simulink model "untitled"  (R2015a)
settings: Solver=ode45  StartTime=0.0  StopTime=10.0  RelTol=1e-3
settings Model: Creator=TaD  LastModifiedBy=TaD

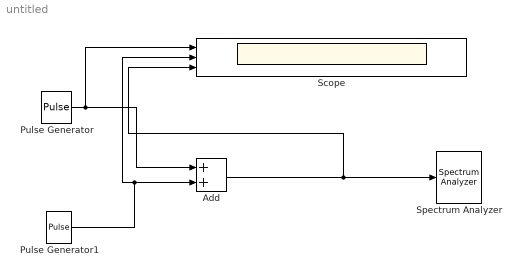
== system untitled ==
  Add : Sum
  Pulse Generator : DiscretePulseGenerator  Amplitude=3  Period=10  PulseWidth=2  VectorParams1D=off
  Pulse Generator1 : DiscretePulseGenerator  PulseType=Time based  Period=10  PulseWidth=5
  Scope : Scope  NumInputPorts=3
      settings: YMin=-5~-5~-5  YMax=5~5~5
  Spectrum Analyzer : SpectrumAnalyzer
  wires:
  Add/1 -> Scope/3, Spectrum Analyzer/1
  Pulse Generator/1 -> Scope/1, Add/1
  Pulse Generator1/1 -> Scope/2, Add/2
